simulink model "chorus"  (R2017a)
settings: Solver=VariableStepAuto  StartTime=0.0  StopTime=inf  RelTol=1e-3
libraries: dspvision x1, dspsrcs4 x1, dspobslib x1, dspsigops x1
settings Model: Creator=ilyas  LastModifiedBy=ilyas

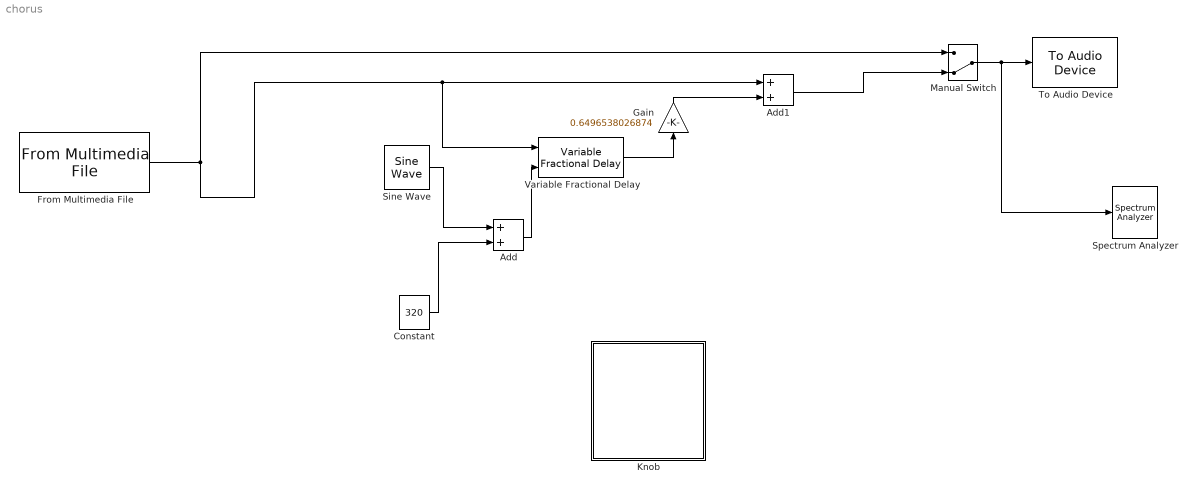
== system chorus ==
  Add : Sum
  Add1 : Sum
  Constant : Constant  Value=320  VectorParams1D=off
  From Multimedia File : dspvision/From Multimedia File  inputFilename=C:\Users\ilyas\Desktop\cours UPMC\Son et image\audio\tpaudio\guitare.wav  loop=on  numPlays=inf  outputStreams=Audio only  videoDataType=single  audioDataType=double  inheritSampleTime=on  userDefinedSampleTime=1/30  noAudioOutput=off  isIntensityVideo=off  fourcc=RGB  colorVideoFormat=Separate color signals  outputEOF=off  dataOrg=Column-major  audioFrameSize=1024  computeAudioFrameSize=off  outSamplingMode=Sample based
      settings: SourceProductBaseCode=VP
  Gain : Gain  Gain=0.6496538026874
  Knob : Subsystem  DialogController=hmiCreateDDGDialog  IsWebBlock=on  mask(MWDashboardBlock){webBlockId=8e0c0283-e84a-4299-8100-d9998a7fb2dd, webBlockType=continuousknob, ShowInLibBrowser=on, ShowInitialText=on, HMISrcModelName=chorus}
      mask prompts: webBlockId "WebBlock Id"; webBlockType "WebBlock Type"; HMISrcModelName "Source Model"
      mask help: SimulinkHMI:dialogs:ContinuousKnobDialogDesc
      mask Help: helpview([docroot '/mapfiles/simulink.map'], 'hmi_knob')
      mask Display:
      | if strcmp(get_param(bdroot(gcb),'BlockDiagramType'), 'library')
      |     image([(matlabroot) '/toolbox/simulink/hmi/icons/ContinuousKnob.png']);
      | end
  Manual Switch : ManualSwitch  CurrentSetting=0
  Sine Wave : dspsrcs4/Sine Wave  Amplitude=80  Frequency=0.7  Phase=0  SampleMode=Discrete  OutComplex=Real  CompMethod=Trigonometric fcn  TableSize=Speed  SampleTime=1/11025  SamplesPerFrame=1024  ResetState=Restart at time zero  OutputFrames=off  dataType=double  wordLen=16  udDataType=sfix(16)  fracBitsMode=Best precision  numFracBits=15  OutDataTypeStr=double  LastOutDataTypeStr=double
  Spectrum Analyzer : SpectrumAnalyzer
  To Audio Device : dspobslib/To Audio Device  deviceName=Default  inheritSampleRate=off  sampleRate=11025  deviceDatatype=Determine from input data type  autoBufferSize=on  bufferSize=4096  queueDuration=1.0  defaultOutputChannelMapping=on  outputChannelMapping=1:2  outputNumUnderrunSamples=off
      settings: SourceProductName=DSP System Toolbox  SourceProductBaseCode=DS
  Variable Fractional Delay : dspsigops/Variable Fractional Delay  mode=OBSOLETE  modeActive=Linear  dmax=10000  InputProcessing=Columns as channels (frame based)  L=4  FarrowL=4  R=10  alpha=1  ic=0  fallbackFIR=Clip to the minimum value necessary for centered kernel  fallbackFarrow=Clip to the minimum value necessary for centered kernel  noDFT=off  roundingMode=Zero  overflowMode=off
      settings: SourceProductName=DSP System Toolbox  SourceProductBaseCode=DS
  wires:
  Constant/1 -> Add/2
  Add/1 -> Variable Fractional Delay/2
  Variable Fractional Delay/1 -> Gain/1
  Gain/1 -> Add1/2
  Sine Wave/1 -> Add/1
  From Multimedia File/1 -> Add1/1, Variable Fractional Delay/1, Manual Switch/1
  Manual Switch/1 -> Spectrum Analyzer/1, To Audio Device/1
  Add1/1 -> Manual Switch/2

== system chorus/Knob ==
